simulink library "nucleoboard_ac_controll_software"  (R2023b)
settings: Solver=VariableStepAuto  StartTime=0.0  StopTime=10.0  RelTol=1e-3
libraries: ac_controller x1, security_block x1, user_interface x1
settings Model: Creator=mueller.chris-it22  LastModifiedBy=kilia

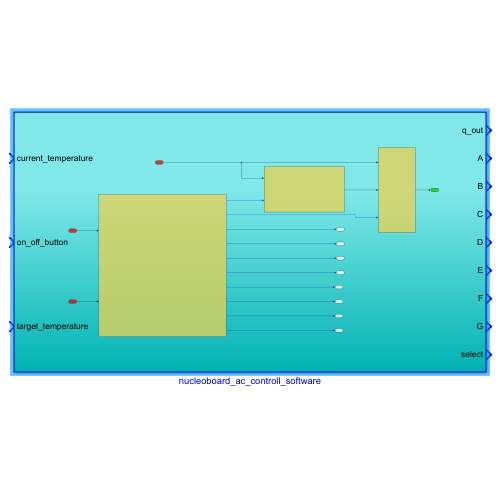
[thumbnail: Simulink's stored preview of the top-level diagram]
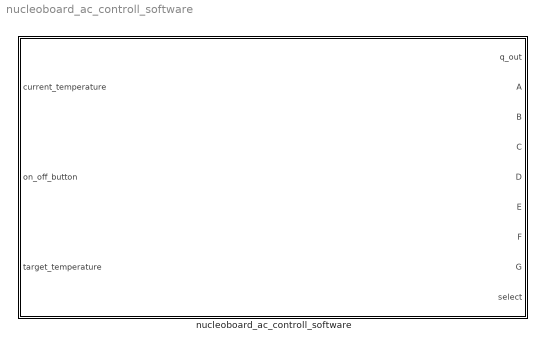
== system nucleoboard_ac_controll_software ==
  nucleoboard_ac_controll_software : Subsystem

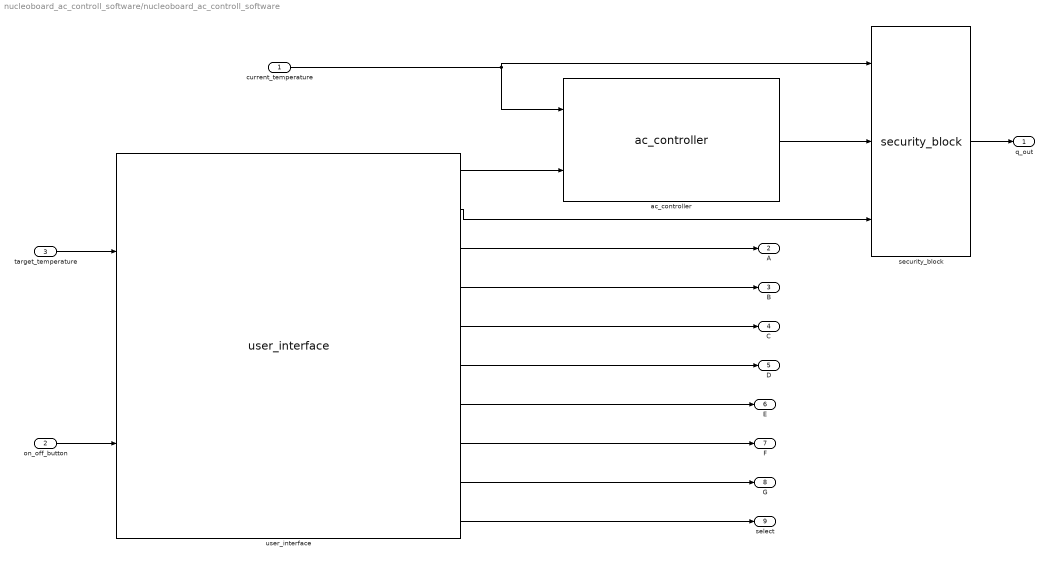
== system nucleoboard_ac_controll_software/nucleoboard_ac_controll_software ==
  current_temperature : Inport
  on_off_button : Inport  Port=2
  target_temperature : Inport  Port=3
  ac_controller : ac_controller/ac_controller  SystemSampleTime=-1  VariantActivationTime=update diagram  AllowFlexibleInterface=on  Latency=0  AutoFrameSizeCalculation=off
  security_block : security_block/security_block  SystemSampleTime=-1  VariantActivationTime=update diagram  AllowFlexibleInterface=on  Latency=0  AutoFrameSizeCalculation=off
  user_interface : user_interface/user_interface  SystemSampleTime=-1  VariantActivationTime=update diagram  AllowFlexibleInterface=on  Latency=0  AutoFrameSizeCalculation=off
  q_out : Outport
  A : Outport  Port=2
  B : Outport  Port=3
  C : Outport  Port=4
  D : Outport  Port=5
  E : Outport  Port=6
  F : Outport  Port=7
  G : Outport  Port=8
  select : Outport  Port=9
  wires:
  current_temperature/1 -> security_block/1, ac_controller/1
  user_interface/2 -> security_block/3
  user_interface/1 -> ac_controller/2
  on_off_button/1 -> user_interface/2
  target_temperature/1 -> user_interface/1
  ac_controller/1 -> security_block/2
  security_block/1 -> q_out/1
  user_interface/3 -> A/1
  user_interface/4 -> B/1
  user_interface/5 -> C/1
  user_interface/6 -> D/1
  user_interface/7 -> E/1
  user_interface/8 -> F/1
  user_interface/9 -> G/1
  user_interface/10 -> select/1
